simulink model "test"  (R2012b)
settings: Solver=ode45  StartTime=0.0  StopTime=10.0  RelTol=1e-3
libraries: simiam x5
settings Model: Creator=samati  LastModifiedBy=samati

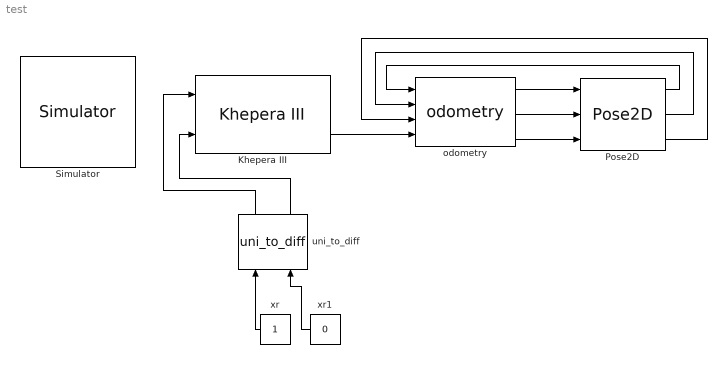
== system test ==
  Khepera III : simiam/Khepera III  x_0=0  y_0=0  theta_0=0  robot_id=1
  Pose2D : simiam/Pose2D  SystemSampleTime=-1
  Simulator : simiam/Simulator  Priority=1
  odometry : simiam/odometry  wheel_radius=r  wheel_base_length=l  ticks_per_rev=2675
  uni_to_diff : simiam/uni_to_diff  wheel_radius=r  wheel_base_length=l
  xr : Constant
  xr1 : Constant  Value=0
  wires:
  Khepera III/2 -> odometry/4
  odometry/1 -> Pose2D/1
  odometry/2 -> Pose2D/2
  odometry/3 -> Pose2D/3
  Pose2D/1 -> odometry/1
  Pose2D/2 -> odometry/2
  Pose2D/3 -> odometry/3
  xr/1 -> uni_to_diff/1
  xr1/1 -> uni_to_diff/2
  uni_to_diff/1 -> Khepera III/1
  uni_to_diff/2 -> Khepera III/2
